simulink model "LQR"  (R2025b)
settings: Solver=VariableStepAuto  StartTime=0.0  StopTime=10.0  RelTol=1e-3
undefined symbols (not defined in the file): A, B, K_LQR_i, K_LQR_x, m, n, xref_lqr
settings Model: Creator=salvo  LastModifiedBy=salvo

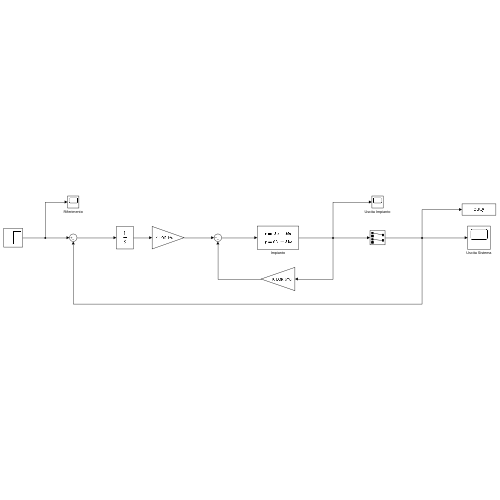
[thumbnail: Simulink's stored preview of the top-level diagram]
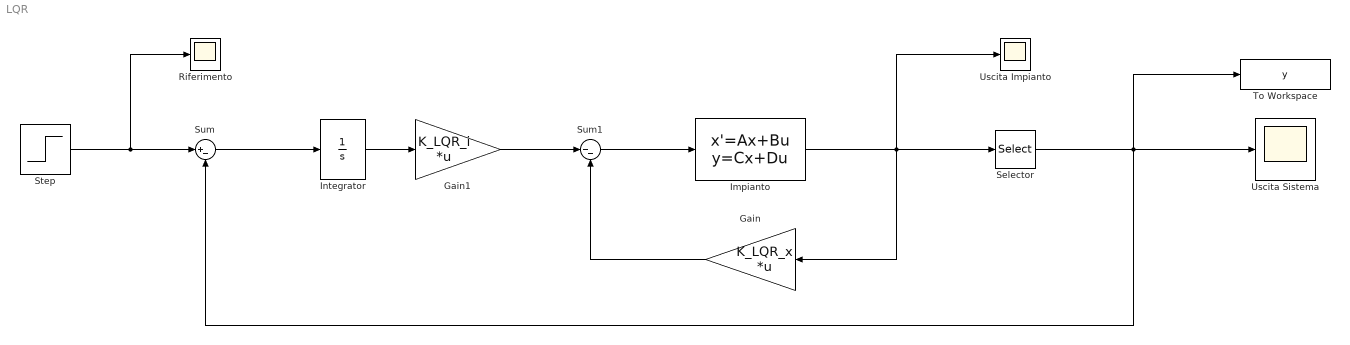
== system LQR ==
  Gain : Gain  Gain=K_LQR_x  Multiplication=Matrix(K*u)
  Gain1 : Gain  Gain=K_LQR_i  Multiplication=Matrix(K*u)
  Impianto : StateSpace  A=A  B=B  C=eye(n)  D=zeros(n,m)  InitialCondition=0
  Integrator : Integrator
  Riferimento : Scope
      settings: ActiveDisplayYMinimum=-0.028675511153547856  ActiveDisplayYMaximum=0.34068834979371876  DataLoggingVariableName=ScopeData2
  Selector : Selector  InputPortWidth=4  IndexOptions=Index vector (dialog)  Indices=[1 3]  OutputSizes=1
  Step : Step  Time=0.0001  After=xref_lqr  SampleTime=0
  Sum : Sum  Inputs=|+-
  Sum1 : Sum  Inputs=|--
  To Workspace : ToWorkspace  VariableName=y  SaveFormat=Timeseries  SampleTime=-1
  Uscita Impianto : Scope
      settings: ActiveDisplayYMinimum=-0.028252708314159585  ActiveDisplayYMaximum=0.25427331686067861
  Uscita Sistema : Scope
      settings: ActiveDisplayYMinimum=-0.033283897184019515  ActiveDisplayYMaximum=0.1723917881632718
  wires:
  Integrator/1 -> Gain1/1
  Gain/1 -> Sum1/2
  Gain1/1 -> Sum1/1
  Sum1/1 -> Impianto/1
  Sum/1 -> Integrator/1
  Step/1 -> Riferimento/1, Sum/1
  Impianto/1 -> Selector/1, Gain/1, Uscita Impianto/1
  Selector/1 -> Sum/2, To Workspace/1, Uscita Sistema/1
